simulink model "motor_hl"  (R2015b)
settings: Solver=FixedStepAuto  StartTime=0.0  StopTime=1000.0  RelTol=1e-3
libraries: arduinolib x2
settings Model: RequirementInfo="{}  %GIDa_e91364bc_06c5_4fa1_9018_e85e8275d570"  SimulationMode=external  ExtModeTrigDuration=2  Creator=Joern  LastModifiedBy=Joern
settings OptimizationCC: OptimizeModelRefInitCode=on  LifeSpan=1  MaxStackSize=64
settings HardwareCC: ProdBitPerInt=16  ProdBitPerPointer=16  ProdLargestAtomicFloat=None  ProdWordSize=8  ProdHWDeviceType=Atmel->AVR
settings ModelReferenceCC: EnableParallelModelReferenceBuilds=on
settings RTWCC: SystemTargetFile=ert.tlc  TemplateMakefile=ert_default_tmf  Description=Embedded Coder  Toolchain=Arduino AVR v1.6.1  BuildConfiguration=Faster Runs
settings CodeAppCC: IgnoreCustomStorageClasses=off
settings ERTTargetCC: GenerateSampleERTMain=on  SupportContinuousTime=on  SupportVariableSizeSignals=on

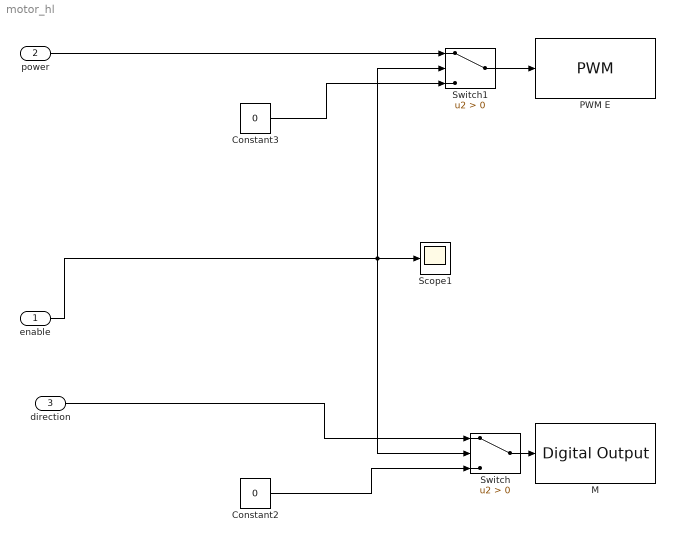
== system motor_hl ==
  enable : Inport
  power : Inport  Port=2
  direction : Inport  Port=3
  Constant2 : Constant  Value=0
  Constant3 : Constant  Value=0
  M : arduinolib/Digital Output  pinNumber=14  blockPlatform=arduino
  PWM E : arduinolib/PWM  pinNumber=8  blockPlatform=arduino
  Scope1 : Scope
  Switch : Switch  Criteria=u2 > Threshold
  Switch1 : Switch  Criteria=u2 > Threshold
  wires:
  Switch/1 -> M/1
  Switch1/1 -> PWM E/1
  enable/1 -> Switch/2, Switch1/2, Scope1/1
  Constant3/1 -> Switch1/3
  direction/1 -> Switch/1
  Constant2/1 -> Switch/3
  power/1 -> Switch1/1
